simulink model "SISO_model"  (R2018b)
settings: Solver=FixedStepAuto  StartTime=0.0  StopTime=Tmod  FixedStep=0.01  RelTol=1e-3
values from neighbouring files (symbols this model uses):
  denominator = FormDenominator(T1, T2, T3, flag)    [Approximation.m]    (also in ApproximationUncertainty.m; BespoiskRegulatorNominal.m = [T1 1]; FormDenominator.m = [T1*T2*T3 T1*T2+T1*T3+T2*T3 T1+T2+T3 1]; Graph1x1.m = handles.savedValueOuMS{2})
  ki = (ro * (Wavt_Ki_rob)) + ((1 - ro) * (Wvsp_Ki_rob))    [MaximumSensitivity1x1.m]    (also in RobAdRegSISO.m = Ki_rob)
  kp = (ro * (Wavt_Kp_rob)) + ((1 - ro) * (Wvsp_Kp_rob))    [MaximumSensitivity1x1.m]    (also in RobAdRegSISO.m = Kp_rob)
  numerator = FormNumerator(k, k2)    [Approximation.m]    (also in ApproximationUncertainty.m; BespoiskRegulatorNominal.m; FormNumerator.m = [k*k_2 k]; Graph1x1.m = handles.savedValueOuMS{1})
  tau = Tauob    (= 0)    [Approximation.m]    (also in ApproximationUncertainty.m = max(tau_array); Graph1x1.m = handles.savedValueOuMS{3}; GraphNom1x1.m = ou11{3}; KombRobReg.m = [tau11 tau12; tau21 tau22])
  Tmod = 500    [Approximation.m]    (also in ApproximationUncertainty.m; Main.m = 100; MainMenu.m = numericValueTmod)
undefined symbols (not defined in the file or in its folder): disturbance1
settings Model: Creator=Asus  LastModifiedBy=stepa

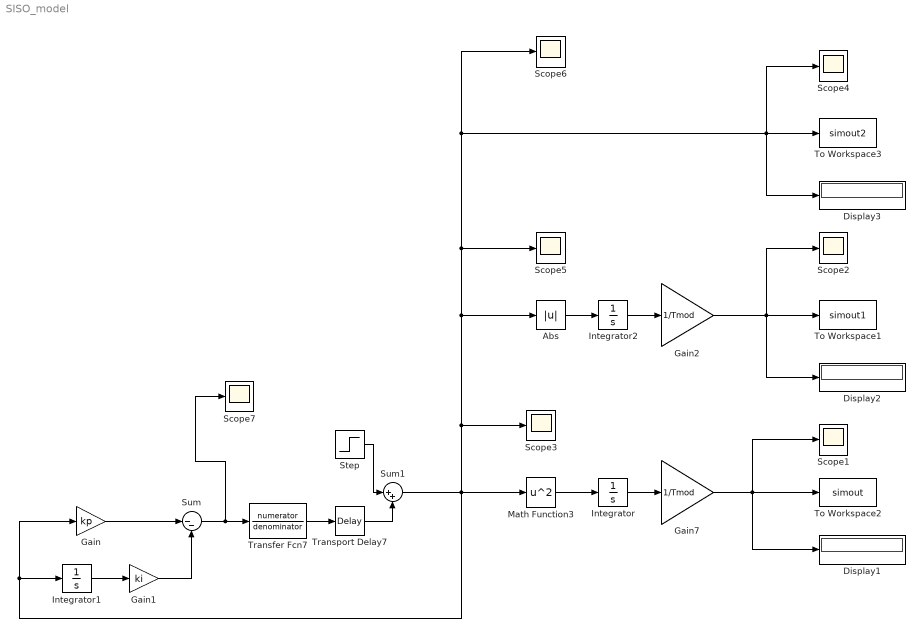
== system SISO_model ==
  Abs : Abs
  Display1 : Display
  Display2 : Display
  Display3 : Display
  Gain : Gain  Gain=kp
  Gain1 : Gain  Gain=ki
  Gain2 : Gain  Gain=1/Tmod
  Gain7 : Gain  Gain=1/Tmod
  Integrator : Integrator
  Integrator1 : Integrator
  Integrator2 : Integrator
  Math Function3 : Math  Operator=square  SaturateOnIntegerOverflow=on
  Scope{1..7} (7 alike) : Scope
  Step : Step  After=disturbance1  SampleTime=0
  Sum : Sum  Inputs=|--
  Sum1 : Sum  Inputs=|++
  To Workspace1 : ToWorkspace  VariableName=simout1  SampleTime=-1
      settings: MaxDataPoints=1
  To Workspace2 : ToWorkspace  VariableName=simout  SampleTime=-1
      settings: MaxDataPoints=1
  To Workspace3 : ToWorkspace  VariableName=simout2  SampleTime=-1
      settings: MaxDataPoints=1
  Transfer Fcn7 : TransferFcn  Numerator=numerator  Denominator=denominator
  Transport Delay7 : TransportDelay  DelayTime=tau
  wires:
  Sum/1 -> Scope7/1, Transfer Fcn7/1
  Transfer Fcn7/1 -> Transport Delay7/1
  Gain/1 -> Sum/1
  Step/1 -> Sum1/1
  Transport Delay7/1 -> Sum1/2
  Math Function3/1 -> Integrator/1
  Integrator/1 -> Gain7/1
  Gain7/1 -> Display1/1, Scope1/1, To Workspace2/1
  Gain2/1 -> Display2/1, Scope2/1, To Workspace1/1
  Integrator2/1 -> Gain2/1
  Abs/1 -> Integrator2/1
  Sum1/1 -> Scope3/1, Scope5/1, Scope6/1, Display3/1, Scope4/1, To Workspace3/1, Abs/1, Integrator1/1, Gain/1, Math Function3/1
  Integrator1/1 -> Gain1/1
  Gain1/1 -> Sum/2
